simulink model "Fig340"  (R2014b)
settings: Solver=ode3  StartTime=0.0  StopTime=5.24288  FixedStep=2e-6  RelTol=1e-5
libraries: commutil2 x1, commrandsrc2 x1
settings Model: Creator=Dennis Silage  LastModifiedBy=Silage
settings DataIOCC: SignalLoggingSaveFormat=ModelDataLogs
settings OptimizationCC: ExpressionDepthLimit=2147483647  InitFltsAndDblsToZero=on
settings DebuggingCC: UnderspecifiedInitializationDetection=Classic  MergeDetectMultiDrivingBlocksExec=none  SolverPrmCheckMsg=none  FcnCallInpInsideContextMsg=UseLocalSettings  StateNameClashWarn=warning
settings GRTTargetCC: CombineOutputUpdateFcns=off  GRTInterface=on

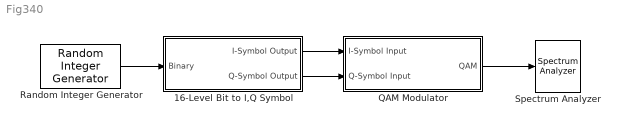
== system Fig340 ==
  16-Level Bit to I,Q Symbol : Subsystem
  QAM Modulator : Subsystem
  Random Integer Generator : commrandsrc2/Random Integer Generator  mul=2  seed=randseed  Ts=1e-3  frameBased=off  sampPerFrame=1  orient=off  outDataType=double
  Spectrum Analyzer : SpectrumAnalyzer
  wires:
  Random Integer Generator/1 -> 16-Level Bit to I,Q Symbol/1(Binary)
  16-Level Bit to I,Q Symbol/1(I-Symbol Output) -> QAM Modulator/1(I-Symbol Input)
  16-Level Bit to I,Q Symbol/2(Q-Symbol Output) -> QAM Modulator/2(Q-Symbol Input)
  QAM Modulator/1(QAM) -> Spectrum Analyzer/1

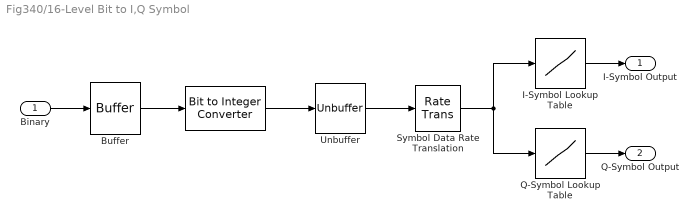
== system Fig340/16-Level Bit to I,Q Symbol ==
  Binary : Inport
  " " : commutil2/Bit to Integer Converter  nbits=4  bitOrder=MSB first  signedOutputValues=Unsigned  outDtype=Inherit via internal rule  outDtypeSigned=Inherit via internal rule
  Buffer : Buffer  N=4  TreatMby1Signals=One channel
  I-Symbol Lookup Table : Lookup_n-D  NumberOfTableDimensions=1  BreakpointsForDimension1=[0,1,2,3,4,5,6,7,8,9,10,11,12,13,14,15]  Table=[-1,-3,-1,-3,1,1,3,3,-1,-1,-3,-3,1,3,1,3]  InternalRulePriority=Speed  RndMeth=Simplest  InputSameDT=on
  Q-Symbol Lookup Table : Lookup_n-D  NumberOfTableDimensions=1  BreakpointsForDimension1=[0,1,2,3,4,5,6,7,8,9,10,11,12,13,14,15]  Table=[1,1,3,3,1,3,1,3,-1,-3,-1,-3,-1,-1,-3,-3]  InternalRulePriority=Speed  RndMeth=Simplest  InputSameDT=on
  Symbol Data Rate Translation : RateTransition  OutPortSampleTime=4e-3
  Unbuffer : Unbuffer  SampleBasedProcessing=Same as frame based
  I-Symbol Output : Outport
  Q-Symbol Output : Outport  Port=2
  wires:
  Symbol Data Rate Translation/1 -> Q-Symbol Lookup Table/1, I-Symbol Lookup Table/1
  Binary/1 -> Buffer/1
  Buffer/1 -> " "/1
  " "/1 -> Unbuffer/1
  Unbuffer/1 -> Symbol Data Rate Translation/1
  I-Symbol Lookup Table/1 -> I-Symbol Output/1
  Q-Symbol Lookup Table/1 -> Q-Symbol Output/1

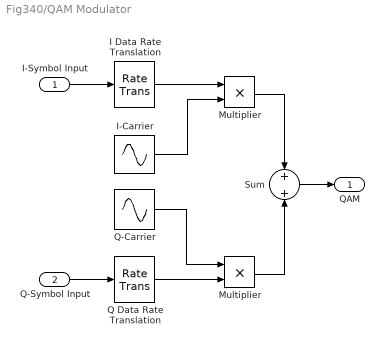
== system Fig340/QAM Modulator ==
  I-Symbol Input : Inport
  Q-Symbol Input : Inport  Port=2
  " Multiplier " : Product  RndMeth=Zero
  I Data Rate Translation : RateTransition  OutPortSampleTime=2e-6
  I-Carrier : Sin  Amplitude=5  Frequency=40000*pi  Phase=pi/2  SampleTime=2e-6  VectorParams1D=off
  Multiplier : Product  RndMeth=Zero
  Q Data Rate Translation : RateTransition  OutPortSampleTime=2e-6
  Q-Carrier : Sin  Amplitude=5  Frequency=40000*pi  SampleTime=2e-6  VectorParams1D=off
  Sum : Sum
  QAM : Outport
  wires:
  I Data Rate Translation/1 -> Multiplier/1
  Q Data Rate Translation/1 -> " Multiplier "/2
  I-Carrier/1 -> Multiplier/2
  Q-Carrier/1 -> " Multiplier "/1
  Multiplier/1 -> Sum/1
  " Multiplier "/1 -> Sum/2
  Sum/1 -> QAM/1
  I-Symbol Input/1 -> I Data Rate Translation/1
  Q-Symbol Input/1 -> Q Data Rate Translation/1
